simulink model "lab3"  (R2023a)
settings: Solver=VariableStepAuto  StartTime=0.0  StopTime=10.0  RelTol=1e-3
settings Model: Creator=mmaji  LastModifiedBy=mmaji

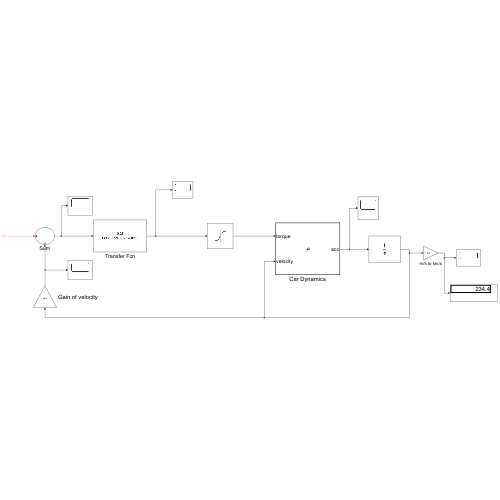
[thumbnail: Simulink's stored preview of the top-level diagram]
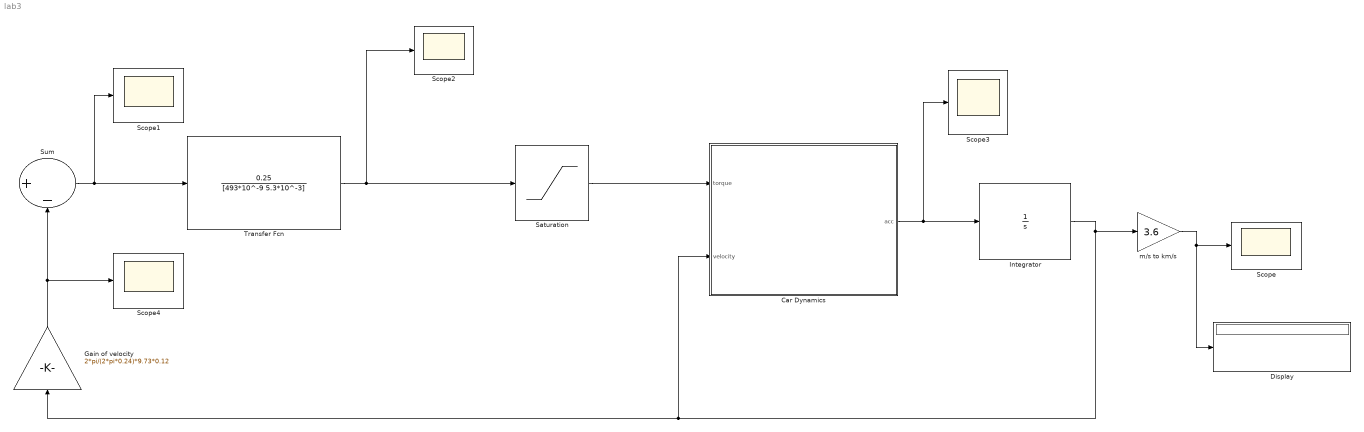
== system lab3 ==
  Car Dynamics : MATLAB Function  TreatAsAtomicUnit=on
  Display : Display
  Gain of velocity : Gain  Gain=2*pi/(2*pi*0.24)*9.73*0.12
  Integrator : Integrator
  Saturation : Saturate  UpperLimit=600  LowerLimit=0
  Scope{,1..4} (5 alike) : Scope
  Sum : Sum  Inputs=|+-
  Transfer Fcn : TransferFcn  Numerator=0.25  Denominator=[493*10^-9 5.3*10^-3]
  m/s to km/s : Gain  Gain=3.6
  wires:
  ? -> Sum/1
  Sum/1 -> Scope1/1, Transfer Fcn/1
  Gain of velocity/1 -> Sum/2, Scope4/1
  Transfer Fcn/1 -> Scope2/1, Saturation/1
  Car Dynamics/1(acc) -> Scope3/1, Integrator/1
  Integrator/1 -> m/s to km/s/1, Gain of velocity/1, Car Dynamics/2(velocity)
  m/s to km/s/1 -> Display/1, Scope/1
  Saturation/1 -> Car Dynamics/1(torque)

== matlab function lab3/Car Dynamics ==
  data: torque input; acc output; velocity input
function acc = fcn( torque, velocity)

acc=(0.6*40.5*torque - 413- 0.3381 *velocity^2)/2100
